simulink library "INT_T50_DD"  (R2016b)
settings: Solver=VariableStepAuto  StartTime=0.0  StopTime=10.0  RelTol=1e-3
settings Model: Creator=guanxiaoxing  LastModifiedBy=guanxiaoxing

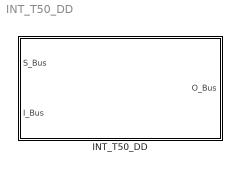
== system INT_T50_DD ==
  INT_T50_DD : Subsystem

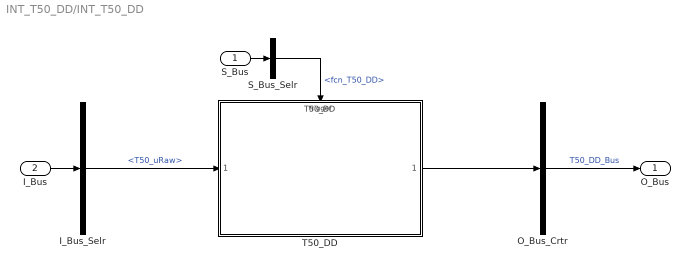
== system INT_T50_DD/INT_T50_DD ==
  S_Bus : Inport
  I_Bus : Inport  Port=2
  I_Bus_Selr : BusSelector  OutputSignals=T50_uRaw
  O_Bus_Crtr : BusCreator  Inputs=1
  S_Bus_Selr : BusSelector  OutputSignals=fcn_T50_DD
  T50_DD : ModelReference  ModelNameDialog=T50_DD  SimulationMode=Normal  ModelReferenceVersion=1.21  TriggerPortName=function  TriggerPortTriggerType=function-call  TriggerPortStatesWhenEnabling=held
  O_Bus : Outport
  wires:
  S_Bus_Selr/1 -> T50_DD/Trigger  "<fcn_T50_DD>"
  S_Bus/1 -> S_Bus_Selr/1
  I_Bus/1 -> I_Bus_Selr/1
  I_Bus_Selr/1 -> T50_DD/1  "<T50_uRaw>"
  O_Bus_Crtr/1 -> O_Bus/1  "T50_DD_Bus"
  T50_DD/1 -> O_Bus_Crtr/1
